simulink model "deadReckoningSim_soln"  (R2023a)
settings: Solver=FixedStepDiscrete  StartTime=0.0  StopTime=200  FixedStep=0.01  RelTol=1e-3
PreLoadFcn:
  | robotParameters;
model workspace (MAT data in the model file):
  axleLength = 0.28
  ticksPerRot = 360
  wheelR = 0.052
undefined symbols (not defined in the file): DiscIntNeverNeededParam, lineLength
libraries: mobileRoboticsTrainingLib x2
settings Model: Creator=sseshadr  LastModifiedBy=minid
settings SolverCC: AlgebraicLoopSolver=TrustRegion
settings DataIOCC: ReturnWorkspaceOutputs=off
settings DebuggingCC: UnconnectedInputMsg=warning  UnconnectedOutputMsg=warning  UnconnectedLineMsg=warning  ArithmeticOperatorsInVariantConditions=warning
settings ModelReferenceCC: EnableRefExpFcnMdlSchedulingChecks=on
settings SFSimCC: SimUseLocalCustomCode=off  CustomCodeUndefinedFunction=UseInterfaceOnly
settings RTWCC: RTWUseLocalCustomCode=off
settings CodeAppCC: StateflowObjectComments=on

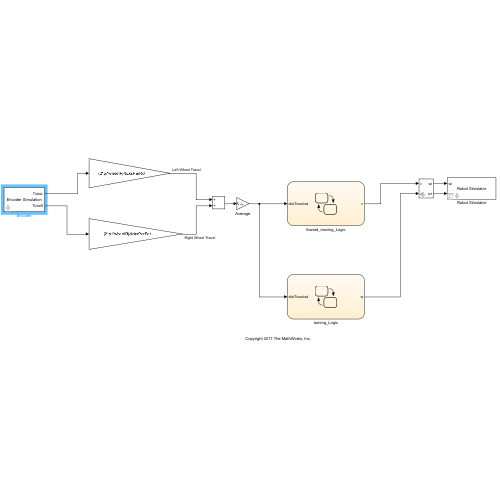
[thumbnail: Simulink's stored preview of the top-level diagram]
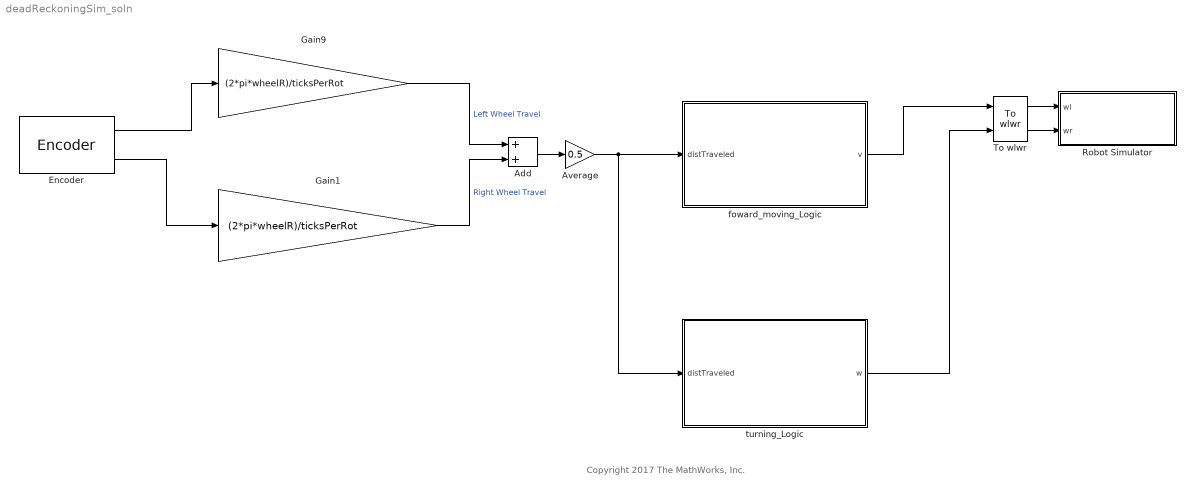
== system deadReckoningSim_soln ==
  note: Copyright 2017 The MathWorks, Inc.
  Add : Sum
  Average : Gain  Gain=0.5
  Encoder : mobileRoboticsTrainingLib/Encoder  axleLength=axleLength  wheelR=wheelR  ticksPerRot=ticksPerRot
      settings: SourceProductName=Mobile Robotics Training Library
  Gain1 : Gain  Gain=(2*pi*wheelR)/ticksPerRot
  Gain9 : Gain  Gain=(2*pi*wheelR)/ticksPerRot
  Robot Simulator : Subsystem  Priority=99  AncestorBlock=mobileRoboticsTrainingLib/Robot Simulator  mask(Robot Simulator){mapVar=[], startX=1, startY=1, startTheta=0, axleLength=axleLength, wheelR=wheelR}
      mask prompts: mapVar "Map Variable"; startX "Start X (m)"; startY "Start Y (m)"; startTheta "Theta (deg)"; axleLength "Axle Length (m)"; wheelR "Wheel Radius (m)"
      mask help: Configure robot simulator to use custom simulation maps and simulate closed-loop mobile robotics systems along with appropriate sensor simulation blocks.
      mask init:
      | set_param(bdroot,'SolverType','Fixed-Step');
      | set_param(bdroot,'Solver','FixedStepDiscrete');
      | 
      | if (exist('Ts'))
      |     set_param(bdroot,'FixedStep','Ts');
      | else
      |     set_param(bdroot,'FixedStep','0.01');
      | end
      | 
      | h = findobj('Name','Robot Simulator');
      | if ~isempty(h)
      |     close (h);
      | end
      | setupRobotSim();
      settings: LibrarySourceBlock=mobileRoboticsTrainingLib/Robot Simulator
      mask Help: web('Robot Simulator.htm')
      mask DialogControl mapCont Prompt: Map Setup
      mask DialogControl initPosCont Prompt: Initial Position
      mask DialogControl setPos Prompt: Set position interactively
      mask DialogControl setPos Callback:
      | %% Set starting point
      | setStartingPoint();
      mask DialogControl initOrientation Prompt: Initial Orientation
      mask DialogControl robotCharCont Prompt: Robot Characteristics
      mask Display: disp('Robot Simulator')
  To wlwr : mobileRoboticsTrainingLib/To wlwr  axleLength=axleLength  wheelR=wheelR
  foward_moving_Logic : Stateflow chart  TreatAsAtomicUnit=on
  turning_Logic : Stateflow chart  TreatAsAtomicUnit=on
  wires:
  Average/1 -> turning_Logic/1(distTraveled), foward_moving_Logic/1(distTraveled)
  foward_moving_Logic/1(v) -> To wlwr/1
  Gain9/1 -> Add/1  "Left Wheel Travel"
  Encoder/2 -> Gain1/1
  Encoder/1 -> Gain9/1
  Add/1 -> Average/1
  Gain1/1 -> Add/2  "Right Wheel Travel"
  To wlwr/1 -> Robot Simulator/1(wl)
  To wlwr/2 -> Robot Simulator/2(wr)
  turning_Logic/1(w) -> To wlwr/2

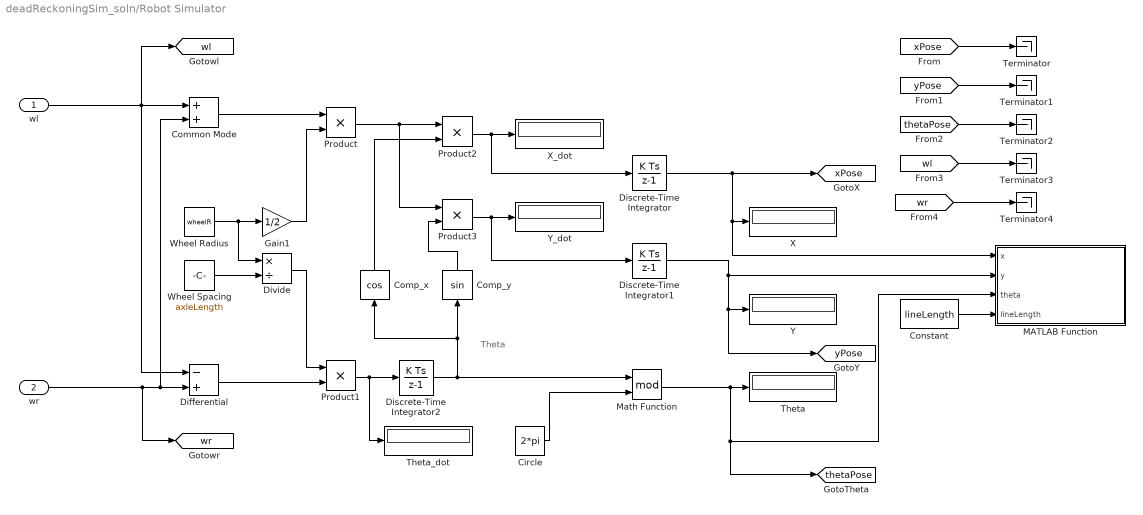
== system deadReckoningSim_soln/Robot Simulator ==
  note: Theta
  wl : Inport
  wr : Inport  Port=2
  Circle : Constant  Value=2*pi
  Common Mode : Sum
  Comp_x : Trigonometry  Operator=cos
  Comp_y : Trigonometry
  Constant : Constant  Value=lineLength
  Differential : Sum  Inputs=-+
  Discrete-Time Integrator : DiscreteIntegrator  InitialCondition=startX  SampleTime=-1  ICPrevOutput=DiscIntNeverNeededParam  ICPrevScaledInput=DiscIntNeverNeededParam
  Discrete-Time Integrator1 : DiscreteIntegrator  InitialCondition=startY  SampleTime=-1  ICPrevOutput=DiscIntNeverNeededParam  ICPrevScaledInput=DiscIntNeverNeededParam
  Discrete-Time Integrator2 : DiscreteIntegrator  InitialCondition=startTheta*(pi/180)  SampleTime=-1  ICPrevOutput=DiscIntNeverNeededParam  ICPrevScaledInput=DiscIntNeverNeededParam
  Divide : Product  Inputs=*/
  Gain1 : Gain  Gain=1/2
  MATLAB Function : MATLAB Function  TreatAsAtomicUnit=on
  Math Function : Math  Operator=mod  SignedPower=on
  Product{,1..3} (4 alike) : Product  RndMeth=Zero
  Terminator{,1..4} (5 alike) : Terminator
  Theta : Display
  Theta_dot : Display
  Wheel Radius : Constant  Value=wheelR
  Wheel Spacing : Constant  Value=axleLength
  X : Display
  X_dot : Display
  Y : Display
  Y_dot : Display
  tag scope: thetaPose=global, wl=global, wr=global, xPose=global, yPose=global
  wires:
  [wr] -> Terminator4/1
  [wl] -> Terminator3/1
  Math Function/1 -> [thetaPose], MATLAB Function/3(theta), Theta/1
  Differential/1 -> Product1/2
  Comp_y/1 -> Product3/2
  Discrete-Time Integrator/1 -> [xPose], MATLAB Function/1(x), X/1
  Product3/1 -> Discrete-Time Integrator1/1, Y_dot/1
  Discrete-Time Integrator1/1 -> Y/1, [yPose], MATLAB Function/2(y)
  Divide/1 -> Product1/1
  wr/1 -> [wr], Common Mode/2, Differential/2
  Discrete-Time Integrator2/1 -> Math Function/1, Comp_x/1, Comp_y/1
  wl/1 -> [wl], Common Mode/1, Differential/1
  Comp_x/1 -> Product2/2
  Product1/1 -> Discrete-Time Integrator2/1, Theta_dot/1
  Wheel Radius/1 -> Divide/1, Gain1/1
  Wheel Spacing/1 -> Divide/2
  Product2/1 -> Discrete-Time Integrator/1, X_dot/1
  Gain1/1 -> Product/2
  Common Mode/1 -> Product/1
  Product/1 -> Product3/1, Product2/1
  Circle/1 -> Math Function/2
  Constant/1 -> MATLAB Function/4(lineLength)
  [xPose] -> Terminator/1
  [yPose] -> Terminator1/1
  [thetaPose] -> Terminator2/1

== matlab function deadReckoningSim_soln/Robot Simulator/MATLAB Function ==
  data: x input; y input; theta input; lineLength input
function plotRobot(x,y,theta,lineLength)
% Get plot details
coder.extrinsic('evalin','plot')
ph1 = evalin('base','PlotHandle1');
ph2 = evalin('base','PlotHandle2');

% Find length orientation line
xp = [x x+lineLength*cos(theta)];
yp = [y y+lineLength*sin(theta)];

% Plot robot
set(ph1,'xdata',xp,'ydata',yp);
set(ph2,'xdata',x,'ydata',y);
drawnow('limitrate')

== stateflow chart deadReckoningSim_soln/turning_Logic ==
  state MoveForward
    entry:
    w = 0;
  state Stop
    entry:
    w = 0.15;
  state stop2
    entry:
    w = 0;
  state Stop1
    entry:
    w = 0.184;
  state stop3
    entry:
    w = 0;
  state Stop2
    entry:
    w = 0.138;
  state stop4
    entry:
    w = 0;
  state Stop3
    entry:
    w = 0.184;
  state stop5
    entry:
    w = 0;
  state Stop4
    entry:
    w = 0.13;
  state stop7
    entry:
    w = 0;
  state Stop5
    entry:
    w = 0.175;
  state stop6
    entry:
    w = 0;
  (default) -> MoveForward : %Start Dead Reckoning
  MoveForward -> Stop : [distTraveled >= 2]
  Stop -> stop2 : [distTraveled>=2.2]
  stop2 -> Stop1 : [distTraveled>=4.2]
  Stop1 -> stop3 : [distTraveled>=4.4]
  stop3 -> Stop2 : [distTraveled >= 6.4]
  Stop2 -> stop4 : [distTraveled>=6.6]
  stop4 -> Stop3 : [distTraveled >= 8.6]
  Stop3 -> stop5 : [distTraveled>=8.8]
  stop5 -> Stop4 : [distTraveled >= 10.8]
  Stop4 -> stop7 : [distTraveled>=11.0]
  stop7 -> Stop5 : [distTraveled >= 13.0]
  Stop5 -> stop6 : [distTraveled>=13.2]
  data: distTraveled input; w output

== stateflow chart deadReckoningSim_soln/foward_moving_Logic ==
  state MoveForward
    entry:
    v = 0.1;
  state Stop
    entry:
    v = 0.0102;
  state stop2
    entry:
    v = 0.1;
  state Stop1
    entry:
    v = 0.0102;
  state stop3
    entry:
    v = 0.1;
  state Stop2
    entry:
    v = 0.0102;
  state stop4
    entry:
    v = 0.1;
  state Stop3
    entry:
    v = 0.0102;
  state stop5
    entry:
    v = 0.1;
  state Stop4
    entry:
    v = 0.0102;
  state stop7
    entry:
    v = 0.1;
  state Stop5
    entry:
    v = 0.0102;
  state stop6
    entry:
    v = 0;
  (default) -> MoveForward : %Start Dead Reckoning
  MoveForward -> Stop : [distTraveled >= 2]
  Stop -> stop2 : [distTraveled>=2.2]
  stop2 -> Stop1 : [distTraveled>=4.2]
  Stop1 -> stop3 : [distTraveled>=4.4]
  stop3 -> Stop2 : [distTraveled >= 6.4]
  Stop2 -> stop4 : [distTraveled>=6.6]
  stop4 -> Stop3 : [distTraveled >= 8.6]
  Stop3 -> stop5 : [distTraveled>=8.8]
  stop5 -> Stop4 : [distTraveled >= 10.8]
  Stop4 -> stop7 : [distTraveled>=11.0]
  stop7 -> Stop5 : [distTraveled >= 12.0]
  Stop5 -> stop6 : [distTraveled>=12.2]
  data: v output; distTraveled input
